simulink model "MSFartoystyring_jallajalla_adaptiv"  (R2019a)
settings: Solver=VariableStepAuto  StartTime=tstart  StopTime=tstop  RelTol=1e-2  EnableMultiTasking=on
undefined symbols (not defined in the file): c, K_d, K_i, K_p, lambda, msfartoystyring, p0, psi0, r0, tsamp, v0
libraries: simulink_extras x1
settings Model: ExtModeAutoUpdateStatusClock=off  Creator=christh  LastModifiedBy=gustavoo
settings DataIOCC: LimitDataPoints=on  SaveFormat=Array  SignalLoggingSaveFormat=ModelDataLogs  ReturnWorkspaceOutputs=off
settings OptimizationCC: ExpressionDepthLimit=2147483647  InitFltsAndDblsToZero=on  LifeSpan=inf
settings DebuggingCC: UnderspecifiedInitializationDetection=Classic  MergeDetectMultiDrivingBlocksExec=none  SolverPrmCheckMsg=warning  FcnCallInpInsideContextMsg=warning  StateNameClashWarn=warning  SFUnexpectedBacktrackingDiag=warning  SFNoUnconditionalDefaultTransitionDiag=warning  ArithmeticOperatorsInVariantConditions=warning
settings HardwareCC: ProdBitPerPointer=32  ProdBitPerSizeT=32  ProdBitPerPtrDiffT=32  ProdLargestAtomicFloat=None  ProdIntDivRoundTo=Undefined  ProdEndianess=Unspecified  ProdWordSize=32  ProdHWDeviceType=32-bit Generic
settings ModelReferenceCC: PropagateSignalLabelsOutOfModel=off
settings SFSimCC: SimUseLocalCustomCode=off
settings RTWCC: RTWUseLocalCustomCode=off
settings CodeAppCC: StateflowObjectComments=on
settings GRTTargetCC: TargetLangStandard=C89/C90 (ANSI)  GeneratePreprocessorConditionals=Disable all  CombineOutputUpdateFcns=off  GRTInterface=on
settings ConfigComp: CovMetricSettings=dw  CovHtmlReporting=on  CovSaveCumulativeToWorkspaceVar=on  CovSaveSingleToWorkspaceVar=on  CovExternalEMLEnable=off

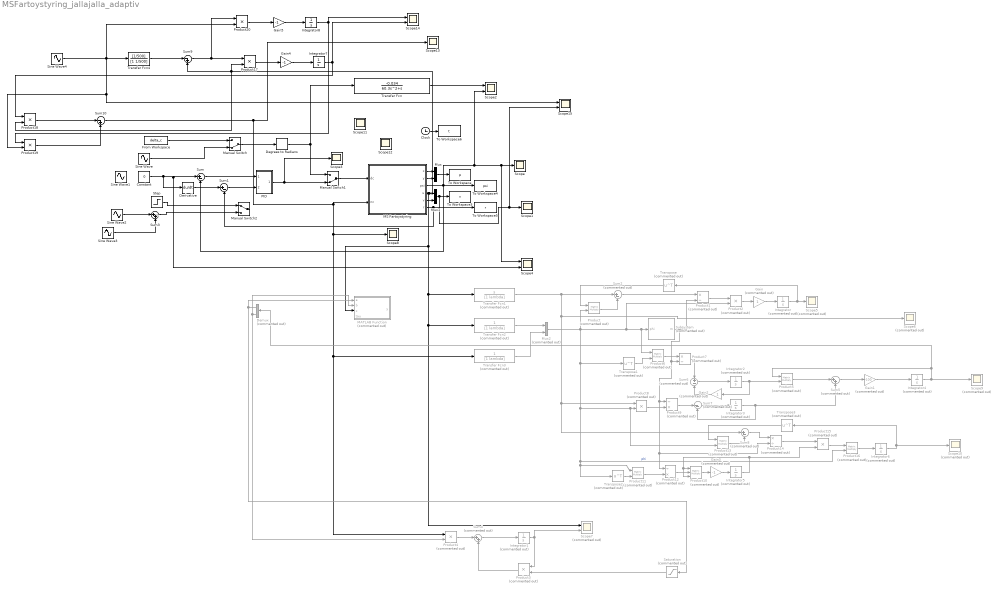
== system MSFartoystyring_jallajalla_adaptiv ==
  note: su,
  Clock : Clock
  Constant : Constant  Value=0
  Degrees to Radians : simulink_extras/Transformations/Degrees to Radians
  Demux : Demux  Commented=on  Outputs=2
  Derivative : Derivative
  From Workspace : FromWorkspace  VariableName=delta_c  SampleTime=0
  Gain : Gain  Commented=on
  Gain1 : Gain  Commented=on  Gain=-100
  Gain2 : Gain  Commented=on
  Gain3 : Gain  Commented=on  Gain=-1
  Gain4 : Gain  Gain=-1
  Gain5 : Gain  Gain=-1
  Integrator : Integrator  Commented=on  InitialCondition=[-10;10]
  Integrator1 : Integrator  Commented=on  InitialCondition=v0(1)
  Integrator2 : Integrator  Commented=on  InitialCondition=[0 0;0 0]
  Integrator3 : Integrator  Commented=on  InitialCondition=[0;0]
  Integrator4 : Integrator  Commented=on  InitialCondition=[-0.1 0.1]  LimitOutput=on  UpperSaturationLimit=[-0.0001 inf]  LowerSaturationLimit=[-inf 0.0001]
  Integrator5 : Integrator  Commented=on  InitialCondition=[100 0; 0 100]
  Integrator6 : Integrator  Commented=on  InitialCondition=[-1; 1]  LimitOutput=on  UpperSaturationLimit=[0; inf]  LowerSaturationLimit=[-inf; 0]
  Integrator7 : Integrator  InitialCondition=5  LimitOutput=on  LowerSaturationLimit=0
  Integrator8 : Integrator  InitialCondition=10  LimitOutput=on  LowerSaturationLimit=0
  MATLAB Function : MATLAB Function  Commented=on  TreatAsAtomicUnit=on
  MS Fartoystyring : Subsystem  mask(MS Fartoystyring for Assignment 3 G&C){x0=p0(1), y0=p0(2), u0=v0(1), v0=v0(2), psi0=psi0, r0=r0, c=c}
      mask prompts: x0 "x(t0) (m)"; y0 "y(t0) (m)"; u0 "u(t0) (m/s)"; v0 "v(t0) (m/s)"; psi0 "psi(t0) (rad)"; r0 "r(t0) (rad/s)"; c "current (0 or 1)"
      mask help:
      | Block corresponding to Figure 1 in the assignment text. Gives the response of the ship.
      |
      | The design speed of MS Fartoystyring is u=8.23 m/s.
      |
      | Input:
      | dc: commanded rudder (rad), dmax=25*pi/180
      | nc: commanded shaft speed (rad/s), nmax=85*2*pi/60
      |
      | Output:
      | x: north pos (m)
      | y: east pos (m)
      | u: surge (m/s)
      | v: sway (m/s)
      | psi: heading (rad)
      | r: yaw (rad/s)
      mask Help: Comments, bugs and help requests can be directed to the TA. Email on course website.
  Manual Switch : ManualSwitch  CurrentSetting=0
  Manual Switch1 : ManualSwitch  CurrentSetting=0
  Manual Switch2 : ManualSwitch
  Mux : Mux  Inputs=2
  Mux1 : Mux  Inputs=2
  Mux2 : Mux  Commented=on  Inputs=2
  PID : Subsystem
  Product{,5..6,11,13,16} (6 alike) : Product  Commented=on  Multiplication=Matrix(*)
  Product1 : Product  Commented=on  Inputs=*/
  Product10 : Product  Commented=on  Inputs=***  Multiplication=Matrix(*)
  Product12 : Product  Commented=on  Inputs=/*
  Product14 : Product  Commented=on  Inputs=*/
  Product{2..4,8,15} (5 alike) : Product  Commented=on
  Product{17..20} (4 alike) : Product
  Product7 : Product  Commented=on  Inputs=*/
  Product9 : Product  Commented=on  Inputs=/*
  Saturation : Saturate  Commented=on  UpperLimit=0  LowerLimit=-inf
  Scope{,1,3,8,11..13} (7 alike) : Scope
  Scope{5..6,9..10} (4 alike) : Scope  Commented=on
  Scope{2,4,14..15} (4 alike) : Scope  NumInputPorts=2
  Scope7 : Scope  Commented=on  NumInputPorts=2
  Sine Wave : Sin  Amplitude=10  Frequency=0.01  SampleTime=0
  Sine Wave1 : Sin  Amplitude=0.4  Frequency=0.004  SampleTime=0
  Sine Wave2 : Sin  Amplitude=2  Bias=2  Frequency=0.0007274  SampleTime=0
  Sine Wave3 : Sin  Amplitude=2.42  Frequency=0.00012425  SampleTime=0
  Sine Wave4 : Sin  Amplitude=2  Bias=4  Frequency=0.001  SampleTime=0
  Step : Step  Before=2  After=4  SampleTime=0
  Subsystem : Subsystem  Commented=on
  Sum : Sum  Inputs=|+-
  Sum1 : Sum  Inputs=|+-
  Sum10 : Sum  Inputs=|-+
  Sum2 : Sum  Commented=on  Inputs=|+-
  Sum3 : Sum  Inputs=|++
  Sum4 : Sum  Commented=on  Inputs=|++
  Sum5 : Sum  Commented=on  Inputs=|++
  Sum6 : Sum  Commented=on  Inputs=+|-
  Sum7 : Sum  Commented=on  Inputs=|--
  Sum8 : Sum  Commented=on  Inputs=|+-
  Sum9 : Sum  Inputs=|-+
  To Workspace : ToWorkspace  VariableName=p  SampleTime=tsamp
  To Workspace3 : ToWorkspace  VariableName=v  SampleTime=tsamp
  To Workspace4 : ToWorkspace  VariableName=psi  SampleTime=tsamp
  To Workspace5 : ToWorkspace  VariableName=r  SampleTime=tsamp
  To Workspace6 : ToWorkspace  VariableName=t  SampleTime=tsamp
  Transfer Fcn : TransferFcn  Numerator=[-0.034]  Denominator=[60.3 1 0]
  Transfer Fcn1 : TransferFcn  Commented=on  Numerator=[1 0]  Denominator=[1 lambda]
  Transfer Fcn2 : TransferFcn  Commented=on  Denominator=[1 lambda]
  Transfer Fcn3 : TransferFcn  Commented=on  Denominator=[1 lambda]
  Transfer Fcn4 : TransferFcn  Numerator=[1/500]  Denominator=[1 1/500]
  Transpose{,1..3} (4 alike) : Math  Commented=on  Operator=transpose  SaturateOnIntegerOverflow=on
  wires:
  Clock/1 -> To Workspace6/1
  MS Fartoystyring/1(x) -> Mux/1
  MS Fartoystyring/2(y) -> Mux/2
  MS Fartoystyring/4(u) -> Scope7/1, Transfer Fcn2/1, Transfer Fcn1/1, MATLAB Function/3(x), Product18/2, Product17/2, Sum9/2, Mux1/1
  MS Fartoystyring/5(v) -> Mux1/2
  Mux/1 -> To Workspace/1
  MS Fartoystyring/6(r) -> Sum1/2, To Workspace5/1
  Degrees to Radians/1 -> Manual Switch1/1, Transfer Fcn/1
  MS Fartoystyring/3(psi) -> Sum/2, To Workspace4/1, Scope2/2, Scope4/1, Scope/1
  Manual Switch/1 -> Degrees to Radians/1
  From Workspace/1 -> Manual Switch/1
  Transfer Fcn/1 -> Scope2/1
  Sine Wave/1 -> Manual Switch/2
  Manual Switch1/1 -> MS Fartoystyring/1(dc)
  PID/1(delta_c) -> Scope3/1, Manual Switch1/2
  Sum/1 -> PID/1(error_psi)
  Constant/1 -> Derivative/1, Scope4/2, Sum/1
  Derivative/1 -> Sum1/1
  Sum1/1 -> PID/2("error_r ")
  Sum10/1 -> Scope13/1, Product4/1, Transfer Fcn3/1, Scope8/1, MS Fartoystyring/2(nc)
  Step/1 -> Manual Switch2/1
  Transfer Fcn2/1 -> Mux2/1
  Transfer Fcn3/1 -> Mux2/2
  Mux2/1 -> Transpose2/1, Product11/1, Product16/2, Product13/2, Product8/2, Transpose1/1, Product6/1, Subsystem/1(phi), Product2/2, Product/2  "phi"
  Transfer Fcn1/1 -> Sum8/1, Product8/1, Scope6/1, Sum2/1
  Product/1 -> Sum2/2
  Sum2/1 -> Product1/1
  Subsystem/1(m) -> Product7/2, Product14/2, Product12/1, Product9/1, Product1/2
  Product1/1 -> Product2/1
  Product2/1 -> Gain/1
  Gain/1 -> Integrator/1
  Integrator/1 -> Scope5/1, Transpose/1
  Sine Wave2/1 -> Sum3/1
  Sine Wave3/1 -> Sum3/2
  Sum3/1 -> Manual Switch2/2
  Sum4/1 -> Integrator1/1
  Product3/1 -> Sum4/2
  Product4/1 -> Sum4/1
  Integrator1/1 -> Scope7/2, Product3/1
  Demux/1 -> MATLAB Function/1(a), Saturation/1
  Demux/2 -> MATLAB Function/2(b), Product4/2
  Saturation/1 -> Product3/2
  Sum5/1 -> Gain1/1
  Gain1/1 -> Integrator4/1
  Integrator2/1 -> Product5/2, Gain2/1
  Product5/1 -> Sum5/1
  Integrator4/1 -> Scope9/1, Demux/1, Product5/1
  Integrator3/1 -> Sum7/2, Sum5/2
  Sum6/1 -> Integrator2/1
  Gain2/1 -> Sum6/2
  Sum7/1 -> Integrator3/1
  Transpose1/1 -> Product6/2
  Product7/1 -> Sum6/1
  Product8/1 -> Product9/2
  Product9/1 -> Sum7/1
  Product6/1 -> Product7/1
  Product10/1 -> Gain3/1
  Integrator5/1 -> Product10/3, Product10/1, Product15/2
  Transpose2/1 -> Product11/2
  Product12/1 -> Product10/2
  Product11/1 -> Product12/2
  Transpose/1 -> Product/1
  Integrator6/1 -> Transpose3/1, Scope10/1
  Transpose3/1 -> Product13/1
  Product13/1 -> Sum8/2
  Sum8/1 -> Product14/1
  Product14/1 -> Product15/1
  Product15/1 -> Product16/1
  Product16/1 -> Integrator6/1
  Gain3/1 -> Integrator5/1
  Mux1/1 -> Scope15/2, Scope1/1, To Workspace3/1
  Transfer Fcn4/1 -> Sum9/1
  Product17/1 -> Gain4/1
  Gain4/1 -> Integrator7/1
  Integrator7/1 -> Scope14/2, Product18/1
  Product18/1 -> Sum10/1
  Product19/1 -> Sum10/2
  Sine Wave4/1 -> Scope15/1, Product19/2, Product20/2, Transfer Fcn4/1
  Sum9/1 -> Product20/1, Product17/1
  Gain5/1 -> Integrator8/1
  Product20/1 -> Gain5/1
  Integrator8/1 -> Scope14/1, Product19/1

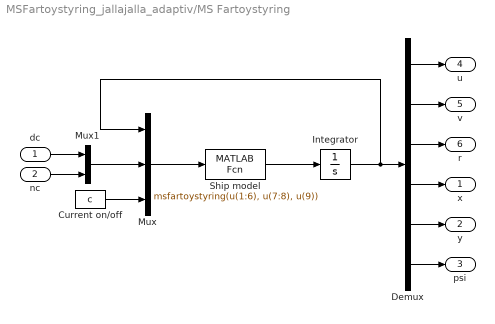
== system MSFartoystyring_jallajalla_adaptiv/MS Fartoystyring ==
  dc : Inport
  nc : Inport  Port=2
  Current on/off : Constant  Value=c
  Demux : Demux  Outputs=6
  Integrator : Integrator  InitialCondition=[u0 v0 r0 x0 y0 psi0]'
  Mux : Mux  Inputs=3
  Mux1 : Mux  Inputs=2
  Ship model : MATLABFcn  MATLABFcn=msfartoystyring(u(1:6), u(7:8), u(9))  OutputDimensions=6
  x : Outport
  y : Outport  Port=2
  psi : Outport  Port=3
  u : Outport  Port=4
  v : Outport  Port=5
  r : Outport  Port=6
  wires:
  Integrator/1 -> Mux/1, Demux/1
  Mux1/1 -> Mux/2
  dc/1 -> Mux1/1
  nc/1 -> Mux1/2
  Demux/1 -> u/1
  Demux/2 -> v/1
  Demux/3 -> r/1
  Demux/4 -> x/1
  Demux/5 -> y/1
  Demux/6 -> psi/1
  Current on/off/1 -> Mux/3
  Ship model/1 -> Integrator/1
  Mux/1 -> Ship model/1

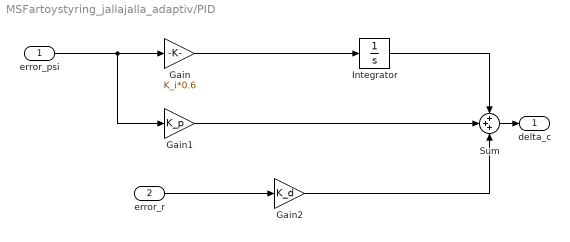
== system MSFartoystyring_jallajalla_adaptiv/PID ==
  error_psi : Inport
  "error_r " : Inport  Port=2
  Gain : Gain  Gain=K_i*0.6
  Gain1 : Gain  Gain=K_p
  Gain2 : Gain  Gain=K_d
  Integrator : Integrator
  Sum : Sum  Inputs=+++
  delta_c : Outport
  wires:
  Gain1/1 -> Sum/2
  error_psi/1 -> Gain1/1, Gain/1
  Gain/1 -> Integrator/1
  Sum/1 -> delta_c/1
  Integrator/1 -> Sum/1
  Gain2/1 -> Sum/3
  "error_r "/1 -> Gain2/1

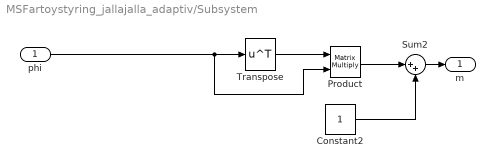
== system MSFartoystyring_jallajalla_adaptiv/Subsystem ==
  phi : Inport
  Constant2 : Constant
  Product : Product  Multiplication=Matrix(*)
  Sum2 : Sum  Inputs=|++
  Transpose : Math  Operator=transpose  SaturateOnIntegerOverflow=on
  m : Outport
  wires:
  phi/1 -> Product/2, Transpose/1
  Transpose/1 -> Product/1
  Product/1 -> Sum2/1
  Sum2/1 -> m/1
  Constant2/1 -> Sum2/2

== matlab function MSFartoystyring_jallajalla_adaptiv/MATLAB Function ==
  data: a input; y output; b input; x input; tau input
function y = adaptive_regulator(a, b, x, tau)
    k = (1/500+a)/b;
    r = -(a-b*k)/b;
y = -k*x+r*tau;
